simulink model "Cardio_Mix_Lange"  (Simulink 7.0)
settings: Solver=ode45  StartTime=0.0  StopTime=10.0  RelTol=1e-3
values from neighbouring files (symbols this model uses):
  PACO2_delayIC = 39.6041    [Cardio_Mix_Lange_IC.m]    (also in Gas_Exchange_IC.m; Respiratory_IC.m = 40.4448)
  PaCO2firstIC = 0.2150    (= 0.215)    [Cardio_Mix_Lange_IC.m]    (also in Gas_Exchange_IC.m; Respiratory_IC.m = -0.2465)
  PaCO2secondIC = 38.4577    [Cardio_Mix_Lange_IC.m]    (also in Gas_Exchange_IC.m; Respiratory_IC.m = 40.3928)
  PAO2_delayIC = 103.8436    [Cardio_Mix_Lange_IC.m]    (also in Gas_Exchange_IC.m; Respiratory_IC.m = 103.1223)
  PaO2firstIC = -0.2838    [Cardio_Mix_Lange_IC.m]    (also in Gas_Exchange_IC.m; Respiratory_IC.m = 0.3557)
  PaO2secondIC = 105.4828    [Cardio_Mix_Lange_IC.m]    (also in Gas_Exchange_IC.m; Respiratory_IC.m = 103.1435)
  T1 = 1    [Cardio_Mix_Lange_IC.m]    (also in Gas_Exchange_IC.m; Respiratory_IC.m)
  T2 = 2    [Cardio_Mix_Lange_IC.m]    (also in Gas_Exchange_IC.m; Respiratory_IC.m)
settings Model: Creator=CLM  LastModifiedBy=CLM
settings OptimizationCC: BlockReduction=off  BooleanDataType=off
settings DebuggingCC: SaveWithParameterizedLinksMsg=none  SignalResolutionControl=TryResolveAllWithWarning  SolverPrmCheckMsg=none  MultiTaskDSMMsg=warning  MultiTaskCondExecSysMsg=none  StrictBusMsg=None
settings HardwareCC: TargetUnknown=on
settings RTWCC: IncludeERTFirstTime=on
settings GRTTargetCC: TargetFcnLib=ansi_tfl_tmw.mat

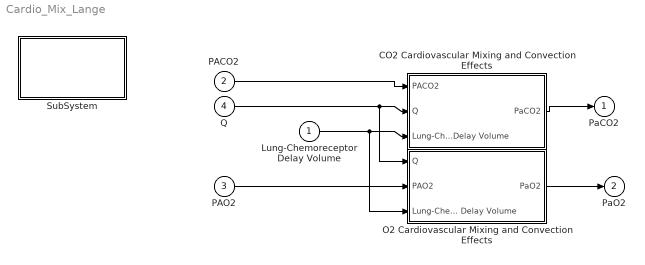
== system Cardio_Mix_Lange ==
  Lung-Chemoreceptor Delay Volume : Inport  OutDataType=sfix(16)  OutScaling=2^0
  PACO2 : Inport  Port=2  OutDataType=sfix(16)  OutScaling=2^0
  PAO2 : Inport  Port=3  OutDataType=sfix(16)  OutScaling=2^0
  Q : Inport  Port=4  OutDataType=sfix(16)  OutScaling=2^0
  CO2 Cardiovascular Mixing and Convection Effects : Subsystem
  O2 Cardiovascular Mixing and Convection Effects : Subsystem
  SubSystem : Subsystem
      settings: OpenFcn=Cardio_Mix_Lange_IC
      mask Display: disp('"double click here"\n to load \nCardio_Mix_Lange \ninitial values');
  PaCO2 : Outport  OutDataType=sfix(16)  OutScaling=2^0
  PaO2 : Outport  Port=2  OutDataType=sfix(16)  OutScaling=2^0
  wires:
  CO2 Cardiovascular Mixing and Convection Effects/1(PaCO2) -> PaCO2/1
  PACO2/1 -> CO2 Cardiovascular Mixing and Convection Effects/1(PACO2)
  Q/1 -> CO2 Cardiovascular Mixing and Convection Effects/2(Q), O2 Cardiovascular Mixing and Convection Effects/1(Q)
  Lung-Chemoreceptor Delay Volume/1 -> CO2 Cardiovascular Mixing and Convection Effects/3(Lung-Chemoreceptor Delay Volume), O2 Cardiovascular Mixing and Convection Effects/3(Lung-Chemoreceptor Delay Volume)
  O2 Cardiovascular Mixing and Convection Effects/1(PaO2) -> PaO2/1
  PAO2/1 -> O2 Cardiovascular Mixing and Convection Effects/2(PAO2)

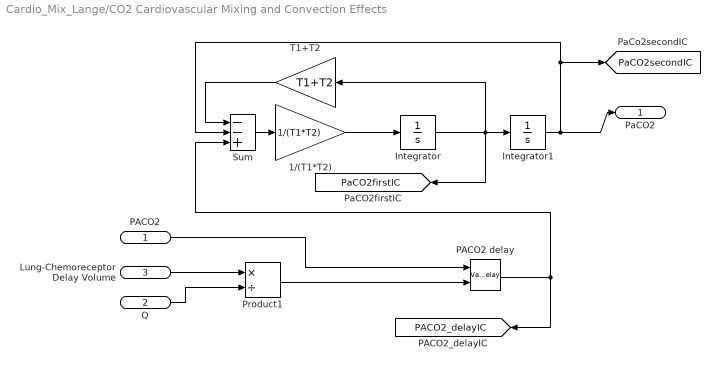
== system Cardio_Mix_Lange/CO2 Cardiovascular Mixing and Convection Effects ==
  PACO2 : Inport  OutDataType=sfix(16)  OutScaling=2^0
  Q : Inport  Port=2  OutDataType=sfix(16)  OutScaling=2^0
  Lung-Chemoreceptor Delay Volume : Inport  Port=3  OutDataType=sfix(16)  OutScaling=2^0
  1/(T1*T2) : Gain  Gain=1/(T1*T2)  ParameterDataType=sfix(16)  ParameterScaling=2^0  OutDataType=sfix(16)  OutScaling=2^0  SaturateOnIntegerOverflow=on
  Integrator : Integrator  InitialCondition=PaCO2firstIC
  Integrator1 : Integrator  InitialCondition=PaCO2secondIC
  PACO2 delay : VariableTransportDelay  MaximumDelay=100  InitialOutput=PACO2_delayIC  MaximumPoints=22528
  Product1 : Product  Inputs=*/  OutDataType=sfix(16)  OutScaling=2^0  SaturateOnIntegerOverflow=on  InputSameDT=on
  Sum : Sum  Inputs=--+  OutDataType=sfix(16)  OutScaling=2^0  SaturateOnIntegerOverflow=on  InputSameDT=on
  T1+T2 : Gain  Orientation=left  Gain=T1+T2  ParameterDataType=sfix(16)  ParameterScaling=2^0  OutDataType=sfix(16)  OutScaling=2^0  SaturateOnIntegerOverflow=on
  PaCO2 : Outport  OutDataType=sfix(16)  OutScaling=2^0
  tag scope: PACO2_delayIC=global, PaCO2firstIC=global, PaCO2secondIC=global
  wires:
  T1+T2/1 -> Sum/1
  Integrator/1 -> T1+T2/1, Integrator1/1, [PaCO2firstIC]
  Sum/1 -> 1/(T1*T2)/1
  1/(T1*T2)/1 -> Integrator/1
  Integrator1/1 -> Sum/2, [PaCO2secondIC], PaCO2/1
  PACO2/1 -> PACO2 delay/1
  PACO2 delay/1 -> [PACO2_delayIC], Sum/3
  Product1/1 -> PACO2 delay/2
  Lung-Chemoreceptor Delay Volume/1 -> Product1/1
  Q/1 -> Product1/2

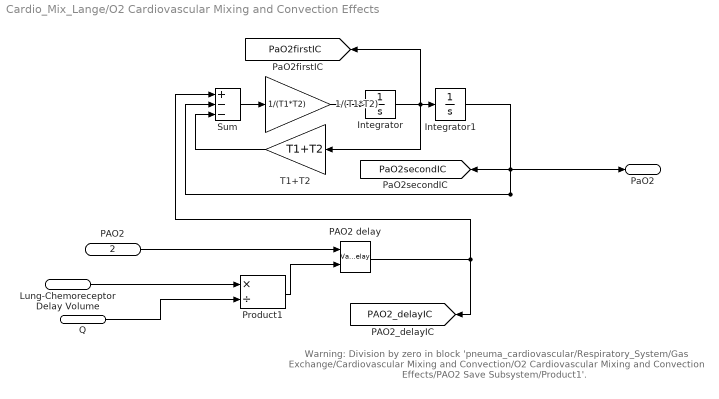
== system Cardio_Mix_Lange/O2 Cardiovascular Mixing and Convection Effects ==
  note: Warning: Division by zero in block 'pneuma_cardiovascular/Respiratory_System/Gas Exchange/Cardiovascular Mixing and Convection/O2 Cardiovascular Mixing and Convection Effects/PAO2 Save Subsystem/Product1'.
  Q : Inport  OutDataType=sfix(16)  OutScaling=2^0
  PAO2 : Inport  Port=2  OutDataType=sfix(16)  OutScaling=2^0
  Lung-Chemoreceptor Delay Volume : Inport  Port=3  OutDataType=sfix(16)  OutScaling=2^0
  1/(T1*T2) : Gain  Gain=1/(T1*T2)  ParameterDataType=sfix(16)  ParameterScaling=2^0  OutDataType=sfix(16)  OutScaling=2^0  SaturateOnIntegerOverflow=on
  Integrator : Integrator  InitialCondition=PaO2firstIC
  Integrator1 : Integrator  InitialCondition=PaO2secondIC
  PAO2 delay : VariableTransportDelay  MaximumDelay=100  InitialOutput=PAO2_delayIC  MaximumPoints=22528
  Product1 : Product  Inputs=*/  OutDataType=sfix(16)  OutScaling=2^0  SaturateOnIntegerOverflow=on  InputSameDT=on
  Sum : Sum  Inputs=+--  OutDataType=sfix(16)  OutScaling=2^0  SaturateOnIntegerOverflow=on  InputSameDT=on
  T1+T2 : Gain  Orientation=left  Gain=T1+T2  ParameterDataType=sfix(16)  ParameterScaling=2^0  OutDataType=sfix(16)  OutScaling=2^0  SaturateOnIntegerOverflow=on
  PaO2 : Outport  OutDataType=sfix(16)  OutScaling=2^0
  tag scope: PAO2_delayIC=global, PaO2firstIC=global, PaO2secondIC=global
  wires:
  1/(T1*T2)/1 -> Integrator/1
  Sum/1 -> 1/(T1*T2)/1
  Integrator/1 -> Integrator1/1, T1+T2/1, [PaO2firstIC]
  Integrator1/1 -> [PaO2secondIC], Sum/2, PaO2/1
  T1+T2/1 -> Sum/3
  Product1/1 -> PAO2 delay/2
  PAO2/1 -> PAO2 delay/1
  PAO2 delay/1 -> [PAO2_delayIC], Sum/1
  Lung-Chemoreceptor Delay Volume/1 -> Product1/1
  Q/1 -> Product1/2

== system Cardio_Mix_Lange/SubSystem ==
